simulink library "cf_lib"  (R2018b)
settings: Solver=VariableStepAuto  StartTime=0.0  StopTime=10.0  RelTol=1e-3
undefined symbols (not defined in the file): inner_maxlim, inner_minlim, inner_thrust_min, swarm, voltage_battery
libraries: $bdroot x1
settings Model: Creator=sebbe  LastModifiedBy=sebbe

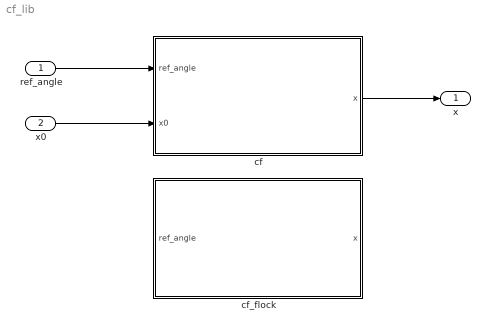
== system cf_lib ==
  ref_angle : Inport  PortDimensions=4
  x0 : Inport  Port=2
  cf : Subsystem
  cf_flock : Subsystem
  x : Outport
  wires:
  ref_angle/1 -> cf/1(ref_angle)
  x0/1 -> cf/2(x0)
  cf/1(x) -> x/1

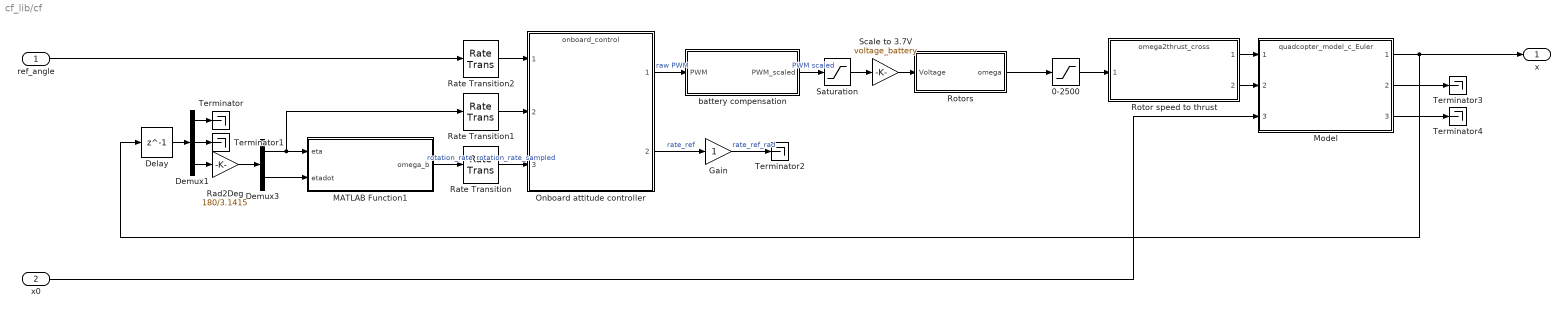
== system cf_lib/cf ==
  ref_angle : Inport  PortDimensions=4
  x0 : Inport  Port=2
  0-2500 : Saturate  UpperLimit=inner_maxlim  LowerLimit=inner_minlim
  Delay : Delay  DelayLength=1  InitialCondition=0
  Demux1 : Demux  Outputs=[3 3 6]
  Demux3 : Demux  Outputs=2
  Gain : Gain
  MATLAB Function1 : MATLAB Function  TreatAsAtomicUnit=on
  Model : ModelReference  ModelNameDialog=quadcopter_model_c_Euler.mdl  ModelReferenceVersion=1.186
  Onboard attitude controller : ModelReference  ModelNameDialog=onboard_control.mdl  ModelReferenceVersion=1.123
  Rad2Deg : Gain  Gain=180/3.1415
  Rate Transition : RateTransition  OutPortSampleTime=inner_rate_h
  Rate Transition1 : RateTransition  OutPortSampleTime=inner_rate_h
  Rate Transition2 : RateTransition  OutPortSampleTime=inner_rate_h
  Rotor speed to thrust : ModelReference  ModelNameDialog=omega2thrust_cross.mdl  ModelReferenceVersion=1.15
  Rotors : Subsystem  TreatAsAtomicUnit=on
  Saturation : Saturate  UpperLimit=1  LowerLimit=inner_thrust_min
  Scale to 3.7V : Gain  Gain=voltage_battery
  Terminator{,1..4} (5 alike) : Terminator
  battery compensation : MATLAB Function  TreatAsAtomicUnit=on
  x : Outport
  wires:
  Saturation/1 -> Scale to 3.7V/1
  Gain/1 -> Terminator2/1  "rate_ref_rad"
  battery compensation/1(PWM_scaled) -> Saturation/1  "PWM scaled"
  Rate Transition2/1 -> Onboard attitude controller/1
  Rate Transition1/1 -> Onboard attitude controller/2
  Rate Transition/1 -> Onboard attitude controller/3  "rotation_rate_sampled"
  x0/1 -> Model/3
  Onboard attitude controller/1 -> battery compensation/1(PWM)  "raw PWM"
  Rotor speed to thrust/2 -> Model/2
  Demux3/1 -> MATLAB Function1/1(eta), Rate Transition1/1
  Demux1/3 -> Rad2Deg/1
  ref_angle/1 -> Rate Transition2/1
  Scale to 3.7V/1 -> Rotors/1(Voltage)
  Rad2Deg/1 -> Demux3/1
  Demux3/2 -> MATLAB Function1/2(etadot)
  Model/1 -> x/1, Delay/1
  0-2500/1 -> Rotor speed to thrust/1
  Demux1/2 -> Terminator1/1
  Model/2 -> Terminator3/1
  Rotor speed to thrust/1 -> Model/1
  MATLAB Function1/1(omega_b) -> Rate Transition/1  "rotation_rate"
  Delay/1 -> Demux1/1
  Model/3 -> Terminator4/1
  Demux1/1 -> Terminator/1
  Rotors/1(omega) -> 0-2500/1
  Onboard attitude controller/2 -> Gain/1  "rate_ref"

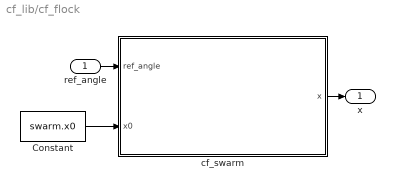
== system cf_lib/cf_flock ==
  ref_angle : Inport
  Constant : Constant  Value=swarm.x0
  cf_swarm : Subsystem  TreatAsAtomicUnit=on
  x : Outport
  wires:
  Constant/1 -> cf_swarm/2(x0)
  cf_swarm/1(x) -> x/1
  ref_angle/1 -> cf_swarm/1(ref_angle)

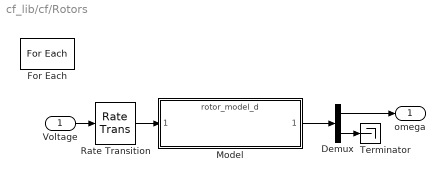
== system cf_lib/cf/Rotors ==
  Voltage : Inport  Partition=on  PartitionDimension=1  PartitionWidth=1  PartitionOffset=0
  Demux : Demux  Outputs=2
  For Each : ForEach  DisableCoverage=on  IndexMode=One-based
  Model : ModelReference  ModelNameDialog=rotor_model_d  ModelReferenceVersion=1.31
  Rate Transition : RateTransition  OutPortSampleTime=continuous_h
  Terminator : Terminator
  omega : Outport  ConcatenationDimension=1
  wires:
  Rate Transition/1 -> Model/1
  Voltage/1 -> Rate Transition/1
  Model/1 -> Demux/1
  Demux/2 -> Terminator/1
  Demux/1 -> omega/1

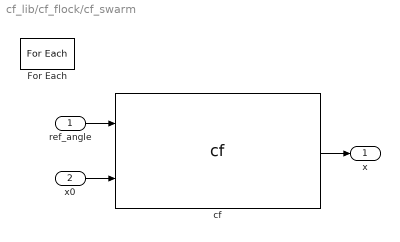
== system cf_lib/cf_flock/cf_swarm ==
  ref_angle : Inport  Partition=on  PartitionDimension=2  PartitionWidth=1  PartitionOffset=0
  x0 : Inport  Port=2  Partition=on  PartitionDimension=2  PartitionWidth=1  PartitionOffset=0
  For Each : ForEach  DisableCoverage=on  IndexMode=One-based
  cf : $bdroot/cf  SystemSampleTime=-1
  x : Outport  ConcatenationDimension=2
  wires:
  ref_angle/1 -> cf/1
  cf/1 -> x/1
  x0/1 -> cf/2

== matlab function cf_lib/cf/MATLAB Function1 ==
  data: eta input; omega_b output; etadot input
function omega_b = etadot2omega_b(eta, etadot)
    % roll(phi) pitch(theta) yaw(psi)
    s_phi = sind(eta(1));
    c_phi = cosd(eta(1));
    s_theta = sind(eta(2));
    c_theta = cosd(eta(2));
    Weta = [1, 0, -s_theta;
        0, c_phi, c_theta*s_phi;
        0, -s_phi, c_theta*c_phi];
    omega_b = Weta*etadot;
end

== matlab function cf_lib/cf/battery compensation ==
  data: PWM input; PWM_scaled output; voltage_battery parameter
function PWM_scaled = bat_comp(PWM, voltage_battery)

c = numel(PWM);
PWM = PWM.*60; % Map to 60g max thrust
PWM = -0.0006239 .* PWM.^2 + 0.088 .* PWM; % Remap to volts
PWM = PWM./voltage_battery; % Get percentage
% Check if over 100%
for i = 1:c
    if PWM(i) > 1
        PWM(i) = 1;
    end
end

% D = D.*65536; % Rescale to uint16
PWM_scaled = PWM;
